simulink model "CoSimV1"  (R2025a)
settings: Solver=FixedStepDiscrete  StartTime=0.0  StopTime=1  FixedStep=Ts_Power  MaxStep=1e-7  RelTol=1e-4  EnableMultiTasking=on
PreLoadFcn:
  | CosimInit
values from neighbouring files (symbols this model uses):
  C_PFC = 2600e-6    (= 0.0026)    [CosimInit.m]
  estimation_src = 3    [CosimInit.m]
  Fnom = 50    [CosimInit.m]
  Fr_I = Fnom*2    (= 100)    [CosimInit.m]
  Ki_V = 80    [CosimInit.m]
  Kp_I = 0.06    [CosimInit.m]
  Kp_V = 0.25    [CosimInit.m]
  Kr_I = 2.5    [CosimInit.m]
  L_PFC = 600e-6    (= 0.0006)    [CosimInit.m]
  Limit_V = 100    [CosimInit.m]
  mm_10cycle_points = mm_points_per_cycle * 10    (= 800)    [CosimInit.m]
  mm_fund_freq = 50    [CosimInit.m]
  mm_points_per_cycle = 80    [CosimInit.m]
  RL_PFC = 20e-3    (= 0.02)    [CosimInit.m]
  Ro = 22.22    [CosimInit.m]
  Ts_Control = 1/Fc    (= 5e-05)    [CosimInit.m]
  Ts_Power = 50e-9    (= 5e-08)    [CosimInit.m]
  use_d_predict = 1    [CosimInit.m]
  use_harmonic = 1    [CosimInit.m]
  use_p_predict = 0    [CosimInit.m]
  Vnom_ac = 240    [CosimInit.m]
undefined symbols (not defined in the file or in its folder): DiscIntNeverNeededParam
libraries: spsSeriesRLCBranchLib x4, spsMeanLib x4, spsCurrentMeasurementLib x3, spsDiodeLib x2, MyLibrary x2, spsFourierLib x2, spsTHDLib x2, pycoexlib x2, simulink x2, spsVoltageMeasurementLib x2, spsACVoltageSourceLib x1, spsIdealSwitchLib x1
settings Model: SimulationMode=accelerator  Creator=The MathWorks, Inc.  LastModifiedBy=changhong
settings SolverCC: AlgebraicLoopSolver=TrustRegion  SolverResetMethod=Robust  AutoInsertRateTranBlk=on
settings DataIOCC: SaveOutput=off  SignalLogging=off  DSMLogging=off  SaveTime=off  ReturnWorkspaceOutputs=off
settings OptimizationCC: LifeSpan=inf
settings DebuggingCC: UnconnectedInputMsg=warning  UnconnectedOutputMsg=warning  UnconnectedLineMsg=warning  SFUnexpectedBacktrackingDiag=warning  SFNoUnconditionalDefaultTransitionDiag=warning  SFExecutionAtInitializationDiag=none  ArithmeticOperatorsInVariantConditions=warning
settings ModelReferenceCC: EnableRefExpFcnMdlSchedulingChecks=on
settings SFSimCC: SimUseLocalCustomCode=off  CustomCodeUndefinedFunction=UseInterfaceOnly
settings RTWCC: RTWUseLocalCustomCode=off  GPUComputeCapability=3.5  DLArmComputeVersion=19.05
settings CodeAppCC: StateflowObjectComments=on
settings GRTTargetCC: TargetLangStandard=C89/C90 (ANSI)
settings ConfigComp: CovMetricSettings=dw  CovSaveCumulativeToWorkspaceVar=on  CovSaveSingleToWorkspaceVar=on  CovExternalEMLEnable=off
settings SimscapeCC: SimscapeNormalizeSystem=off  SimscapeNominalValues={1, 'bar'; 1, 'cm^3/s'; 1, 'bar*kg/s'; 1, 'kJ/kg'; 1, 'kW'; }

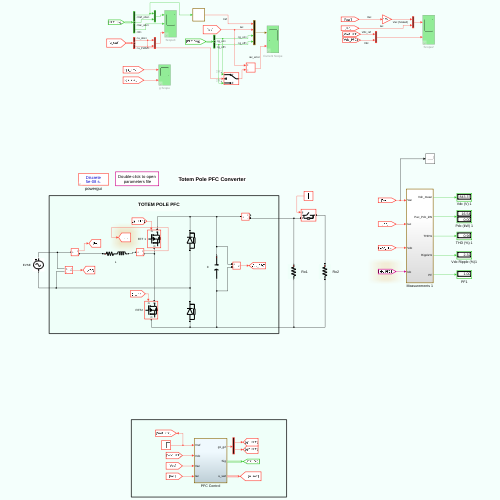
[thumbnail: Simulink's stored preview of the top-level diagram]
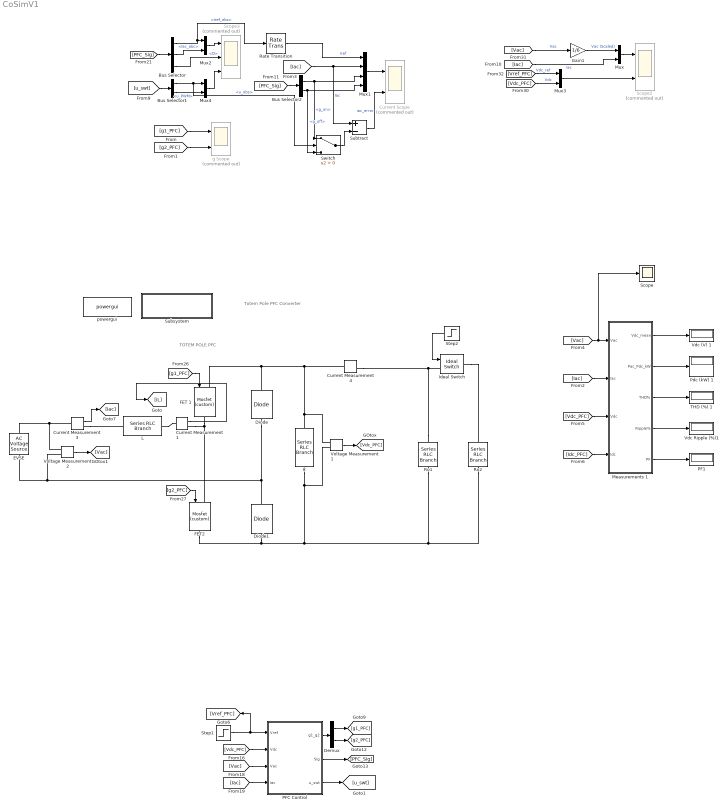
== system CoSimV1 ==
  note: Totem Pole PFC Converter
  note: TOTEM POLE PFC
  Bus Selector : BusSelector  OutputSignals=Iref_obs,Iac_abc,D
  Bus Selector1 : BusSelector  OutputSignals=u_obs,u_PWM
  Bus Selector2 : BusSelector  OutputSignals=g_on,g_off
  C : spsSeriesRLCBranchLib/Series RLC Branch  LConnTagsString=__new0  RConnTagsString=__new0  BranchType=C  Resistance=1  Inductance=1e-3  SetiL0=off  InitialCurrent=0  Capacitance=C_PFC  Setx0=on  InitialVoltage=375  Measurements=None
  Current Measurement1 : spsCurrentMeasurementLib/Current Measurement  PhasorSimulation=off  OutputType=Complex  PSBequivalent=0
  Current Measurement3 : spsCurrentMeasurementLib/Current Measurement  PhasorSimulation=off  OutputType=Complex  PSBequivalent=0
  Current Measurement4 : spsCurrentMeasurementLib/Current Measurement  PhasorSimulation=off  OutputType=Complex  PSBequivalent=0
  Current Scope : Scope  Commented=on  NumInputPorts=2
      settings: ActiveDisplayYMinimum=-76.387109863432016  ActiveDisplayYMaximum=79.51420484932207  DataLoggingVariableName=ScopeData3
  Demux : Demux  Outputs=2
  Diode : spsDiodeLib/Diode  Ron=Ron_Diode  Lon=0  Vf=Vf  IC=0  UseSnubber=0  Rs=1e6  Cs=inf  Measurements=off
  Diode1 : spsDiodeLib/Diode  Ron=Ron_Diode  Lon=0  Vf=Vf  IC=0  UseSnubber=0  Rs=1e6  Cs=inf  Measurements=off
  EVSE : spsACVoltageSourceLib/AC Voltage Source  Amplitude=Vnom_ac*sqrt(2)  Phase=0  Frequency=Fnom  SampleTime=Ts_Power  Measurements=None  BusType=swing  Pref=10e3  Qref=0  Qmin=-inf  Qmax=+inf
  FET 1 : MyLibrary/Mosfet (custom)  Ron=Ron_FET  Lon=0  Rd=Ron_Diode  Vfd=Vf  IC=0  Rs=1e6  Cs=inf  Measurements=off
  FET2 : MyLibrary/Mosfet (custom)  Ron=Ron_FET  Lon=0  Rd=Ron_Diode  Vfd=Vf  IC=0  Rs=1e6  Cs=inf  Measurements=off
  Gain1 : Gain  Gain=1/6
  Ideal Switch : spsIdealSwitchLib/Ideal Switch  Ron=0.001  Lon=0  IC=0  Rs=1e5  Cs=inf  Measurements=off
  L : spsSeriesRLCBranchLib/Series RLC Branch  LConnTagsString=__new0  RConnTagsString=__new0  BranchType=RL  Resistance=RL_PFC  Inductance=L_PFC  SetiL0=off  InitialCurrent=0  Capacitance=1e-6  Setx0=off  InitialVoltage=0  Measurements=None
  Measurements 1 : Subsystem
  Mux{,2..4} (4 alike) : Mux  Inputs=2
  Mux1 : Mux
  PF1 : Display
      settings: Format=bank  Decimation=100
  PFC Control : Subsystem
  Pdc (kW) 1 : Display
      settings: Format=bank  Decimation=100
  Rate Transition : RateTransition
  Ro1 : spsSeriesRLCBranchLib/Series RLC Branch  LConnTagsString=__new0  RConnTagsString=__new0  BranchType=R  Resistance=Ro*2  Inductance=200e-6  SetiL0=off  InitialCurrent=0  Capacitance=400e-6  Setx0=off  InitialVoltage=0  Measurements=None
  Ro2 : spsSeriesRLCBranchLib/Series RLC Branch  LConnTagsString=__new0  RConnTagsString=__new0  BranchType=R  Resistance=Ro*2  Inductance=200e-6  SetiL0=off  InitialCurrent=0  Capacitance=400e-6  Setx0=off  InitialVoltage=0  Measurements=None
  Scope : Scope
      settings: DataLoggingVariableName=ScopeData7
  Scope2 : Scope  Commented=on  NumInputPorts=2
      settings: ActiveDisplayYMinimum=-127.22187930583854  ActiveDisplayYMaximum=127.21088523305926  DataLoggingVariableName=ScopeData11
  Scope3 : Scope  Commented=on  NumInputPorts=3
      settings: ActiveDisplayYMinimum=-13.42740578837777  ActiveDisplayYMaximum=110.84665209539996  DataLoggingVariableName=ScopeData2
  Step1 : Step  Time=0.2  Before=350  After=400  SampleTime=Ts_Power
  Step2 : Step  Time=0.4  SampleTime=Ts_Power
  Subsystem : Subsystem
      settings: OpenFcn=edit('Totem_Pole_PFC_v1_data');
      mask Display: disp('Double-click to open\n parameters file');
  Subtract : Sum  Inputs=+-
  Switch : Switch  Criteria=u2 > Threshold  SaturateOnIntegerOverflow=off  InputSameDT=off
  THD (%) 1 : Display
      settings: Format=bank  Decimation=100
  Vdc (V) 1 : Display
      settings: Format=bank  Decimation=100
  Vdc Ripple (%)1 : Display
      settings: Format=bank  Decimation=100
  Voltage Measurement1 : spsVoltageMeasurementLib/Voltage Measurement  PhasorSimulation=off  OutputType=Complex  PSBequivalent=0
  Voltage Measurement2 : spsVoltageMeasurementLib/Voltage Measurement  PhasorSimulation=off  OutputType=Complex  PSBequivalent=0
  g Scope : Scope  Commented=on  NumInputPorts=2
      settings: ActiveDisplayYMinimum=-0.12499999999999997  ActiveDisplayYMaximum=1.125
  powergui : spspowerguiLib/powergui  Priority=1  SimulationMode=Discrete  SampleTime=Ts_Power  frequency=60  Iterations=50  frequencyindice=0  Pbase=100e6  ErrMax=1e-4  UnitsV=kV  UnitsW=MW  buscounter=0  FunctionMessages=off  echomessages=off  EnableUseOfTLC=off  CurrentSourceSwitches=off  DisableSnubberDevices=off  DisableRonSwitches=off  DisableVfSwitches=off  DisplayEquations=off  AutomaticDiscreteSolvers=off  SolverType=Tustin/Backward Euler (TBE)  Interpol=off  ExternalGateDelay=off  methode=off  Ts=100  x0status=blocks  SPID=on  SwTol=0  HookPort=off  NonlinearTolerance=1e-4  nMaxIteration=100  ContinueOnMaxIteration=off  RestoreLinks=warning  ResistiveCurrentMeasurement=off  Frange=[0:2:500]  Ylog=off  Xlog=on  ShowGrid=off  save=off  variable=ZData  structure=0  ZoomFFT=off  StartTime=0.0  cycles=1  DisplayStyle=1  fundamental=60  FreqAxis=off  MaxFrequency=1000  frequencyindicesteady=1  RmsSteady=1  display=off
  wires:
  Current Measurement3/1 -> [Iac]
  [g1_PFC] -> FET 1/1
  [g2_PFC] -> FET2/1
  Voltage Measurement1/1 -> [Vdc_PFC]
  Step2/1 -> Ideal Switch/1
  Voltage Measurement2/1 -> [Vac]
  Current Measurement1/1 -> [iL]
  Step1/1 -> PFC Control/1(Vref), [Vref_PFC]
  Demux/1 -> [g1_PFC]
  Demux/2 -> [g2_PFC]
  Switch/1 -> Subtract/2
  Bus Selector/1 -> Rate Transition/1, Mux2/1  "<Iref_obs>"
  Rate Transition/1 -> Mux1/1  "Iref"
  Bus Selector1/1 -> Mux4/1, Switch/2  "<u_obs>"
  Bus Selector/2 -> Mux2/2  "<Iac_abc>"
  Mux3/1 -> Scope2/2
  Mux/1 -> Scope2/1
  [g2_PFC] -> g Scope/2
  Bus Selector2/2 -> Mux1/4, Switch/3  "<g_off>"
  Measurements 1/5(PF) -> PF1/1
  [Idc_PFC] -> Measurements 1/4(Idc)
  Bus Selector1/2 -> Mux4/2  "<u_PWM>"
  [Vac] -> Gain1/1  "Vac"
  Measurements 1/2(Pac_Pdc_kW) -> Pdc (kW) 1/1
  Bus Selector/3 -> Scope3/2  "<D>"
  Measurements 1/4(Ripple%) -> Vdc Ripple (%)1/1
  [u_swt] -> Bus Selector1/1
  Mux1/1 -> Current Scope/1
  Gain1/1 -> Mux/1  "Vac (Scaled)"
  [PFC_Sig] -> Bus Selector2/1
  [g1_PFC] -> g Scope/1
  [Vdc_PFC] -> Measurements 1/3(Vdc)
  Measurements 1/3(THD%) -> THD (%) 1/1
  [Iac] -> Subtract/1, Mux1/2  "Iac"
  [Vac] -> Scope/1, Measurements 1/1(Vac)
  [Iac] -> Mux/2  "Iac"
  [PFC_Sig] -> Bus Selector/1
  Measurements 1/1(Vdc_mean) -> Vdc (V) 1/1
  [Iac] -> Measurements 1/2(Iac)
  Bus Selector2/1 -> Switch/1, Mux1/3  "<g_on>"
  Mux2/1 -> Scope3/1
  [Vref_PFC] -> Mux3/1  "Vdc_ref"
  [Vdc_PFC] -> Mux3/2  "Vdc"
  Mux4/1 -> Scope3/3
  Subtract/1 -> Current Scope/2  "iac_error"
  [Vdc_PFC] -> PFC Control/2(Vdc)
  [Vac] -> PFC Control/3(Vac)
  [Iac] -> PFC Control/4(Iac)
  PFC Control/1(g1_g2) -> Demux/1
  PFC Control/2(Sig) -> [PFC_Sig]
  PFC Control/3(u_swt) -> [u_swt]
  connections:
  Ro1/RConn1 -- C/RConn1 -- Voltage Measurement1/LConn2 -- FET2/RConn1 -- Diode1/LConn1 -- Ro2/RConn1
  FET2/LConn1 -- FET 1/RConn1 -- Current Measurement1/RConn1
  EVSE/LConn1 -- Diode/LConn1 -- Diode1/RConn1 -- Voltage Measurement2/LConn2
  Diode/RConn1 -- FET 1/LConn1 -- Voltage Measurement1/LConn1 -- C/LConn1 -- Current Measurement4/LConn1
  Ro1/LConn1 -- Current Measurement4/RConn1 -- Ideal Switch/LConn1
  EVSE/RConn1 -- Current Measurement3/LConn1 -- Voltage Measurement2/LConn1
  L/RConn1 -- Current Measurement1/LConn1
  Current Measurement3/RConn1 -- L/LConn1
  Ideal Switch/RConn1 -- Ro2/LConn1

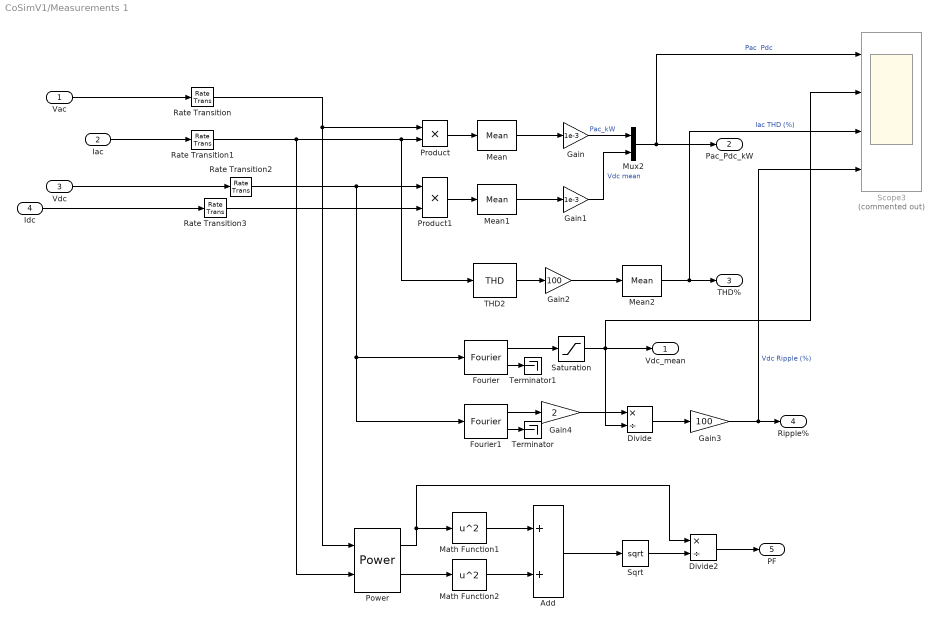
== system CoSimV1/Measurements 1 ==
  Vac : Inport
  Iac : Inport  Port=2
  Vdc : Inport  Port=3
  Idc : Inport  Port=4
  Add : Sum
  Divide : Product  Inputs=*/
  Divide2 : Product  Inputs=*/
  Fourier : spsFourierLib/Fourier  Freq=Fnom  n=0  InInit=[0, 0]  Ts=Ts_Control
  Fourier1 : spsFourierLib/Fourier  Freq=Fnom  n=2  InInit=[0, 0]  Ts=Ts_Control
  Gain : Gain  Gain=1e-3
  Gain1 : Gain  Gain=1e-3
  Gain2 : Gain  Gain=100
  Gain3 : Gain  Gain=100
  Gain4 : Gain  Gain=2
  Math Function1 : Math  Operator=square
  Math Function2 : Math  Operator=square
  Mean : spsMeanLib/Mean  Freq=Fnom  Vinit=0  Ts=Ts_Control
  Mean1 : spsMeanLib/Mean  Freq=Fnom  Vinit=0  Ts=Ts_Control
  Mean2 : spsMeanLib/Mean  Freq=Fnom  Vinit=0  Ts=Ts_Control
  Mux2 : Mux  Inputs=2
  Power : spsPowerLib/Power  Freq=Fnom  Vinit=[1, 0]  Iinit=[1, 0]  Ts=Ts_Control
  Product : Product
  Product1 : Product
  Rate Transition{,1..3} (4 alike) : RateTransition  OutPortSampleTime=Ts_Control
  Saturation : Saturate  UpperLimit=inf  LowerLimit=eps
  Scope3 : Scope  Commented=on  NumInputPorts=4
      settings: ActiveDisplayYMinimum=-1.32447  ActiveDisplayYMaximum=11.92024
  Sqrt : Sqrt
  THD2 : spsTHDLib/THD  Freq=Fnom  Ts=Ts_Control
  Terminator : Terminator
  Terminator1 : Terminator
  Vdc_mean : Outport
  Pac_Pdc_kW : Outport  Port=2
  THD% : Outport  Port=3
  Ripple% : Outport  Port=4
  PF : Outport  Port=5
  wires:
  Gain1/1 -> Mux2/2  "Vdc mean"
  Product1/1 -> Mean1/1
  Mean/1 -> Gain/1
  Product/1 -> Mean/1
  Gain/1 -> Mux2/1  "Pac_kW"
  THD2/1 -> Gain2/1
  Mean1/1 -> Gain1/1
  Iac/1 -> Rate Transition1/1
  Mux2/1 -> Scope3/1, Pac_Pdc_kW/1  "Pac  Pdc"
  Gain2/1 -> Mean2/1
  Mean2/1 -> Scope3/3, THD%/1  "Iac THD (%)"
  Fourier/2 -> Terminator1/1
  Fourier/1 -> Saturation/1
  Saturation/1 -> Scope3/2, Vdc_mean/1, Divide/2
  Divide/1 -> Gain3/1
  Fourier1/1 -> Gain4/1
  Gain4/1 -> Divide/1
  Fourier1/2 -> Terminator/1
  Gain3/1 -> Scope3/4, Ripple%/1  "Vdc Ripple (%)"
  Power/1 -> Math Function1/1, Divide2/1
  Power/2 -> Math Function2/1
  Math Function1/1 -> Add/1
  Math Function2/1 -> Add/2
  Add/1 -> Sqrt/1
  Sqrt/1 -> Divide2/2
  Divide2/1 -> PF/1
  Rate Transition1/1 -> Power/2, THD2/1, Product/2
  Vdc/1 -> Rate Transition2/1
  Idc/1 -> Rate Transition3/1
  Rate Transition/1 -> Power/1, Product/1
  Vac/1 -> Rate Transition/1
  Rate Transition2/1 -> Product1/1, Fourier/1, Fourier1/1
  Rate Transition3/1 -> Product1/2

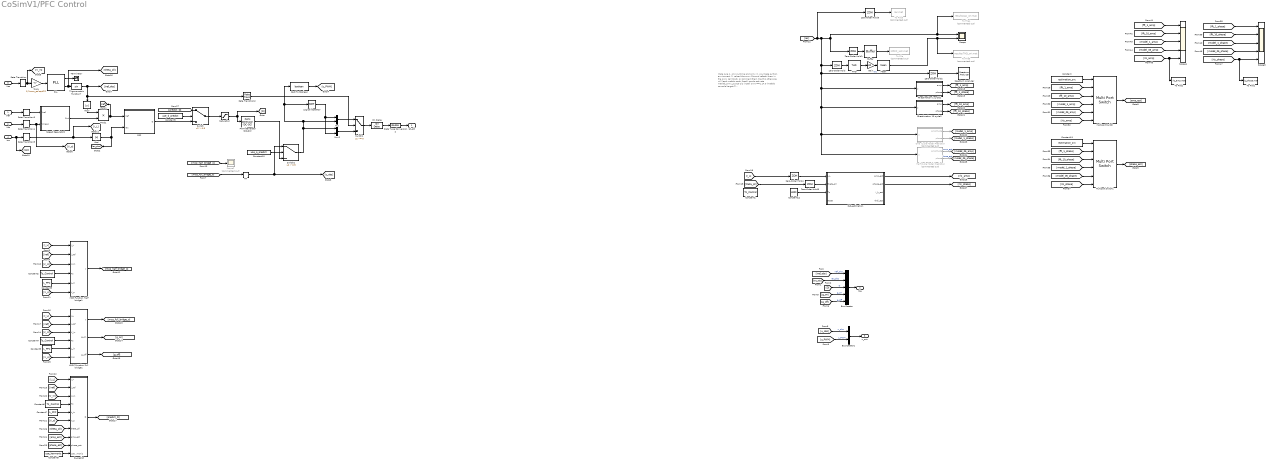
== system CoSimV1/PFC Control ==
  note: Make sure
      | 1. onnxruntime and onnx in your base python enviroment.
      | 2. reload the onnx file and refresh them in the onnx call block.
      | or comment them like this
      | otherwise will lead matlab crash
      |
      | (bash)
      | conda activate matlab_onnx_py310
      | pip install onnx==1.14.0
      |
      | (matlab console)
      | target = "/home/changhong/anaconda3/envs/matlab_onnx_py310/bin/python";
      | pe = pyenv
      | pyenv("Version", target)
  Vref : Inport
  Vdc : Inport  Port=2
  Vac : Inport  Port=3
  Iac : Inport  Port=4
  AbsI : Abs  SaturateOnIntegerOverflow=off
  AbsV : Abs  SaturateOnIntegerOverflow=off
  Buffer : Buffer  N=80  V=79  OutputFrames=off
  Bus Creator : BusCreator  Inputs=5
  Bus Creator1 : BusCreator  Inputs=2
  Cast To Boolean : DataTypeConversion  OutDataTypeStr=boolean  SaturateOnIntegerOverflow=off  RndMeth=Floor
  Constant : Constant  Value=estimation_src
  Constant{1..2,4,6} (4 alike) : Constant  Value=Ts_Control
  Constant10 : Constant  Value=use_p_predict
  Constant11 : Constant  Value=estimation_src
  Constant12 : Constant  Value=4000
  Constant3 : Constant  Value=L_PFC
  Constant5 : Constant  Value=L_PFC
  Constant7 : Constant  Value=L_PFC
  Constant8 : Constant  Value=use_harmonic
  Constant9 : Constant  Value=use_d_predict
  D_predict : MATLAB Function  TreatAsAtomicUnit=on
  Data Type Conversion2 : DataTypeConversion  OutDataTypeStr=double  SaturateOnIntegerOverflow=off  RndMeth=Floor
  Gain : Gain  Gain=100
  Half Cycle Model Prediction : Subsystem  Commented=on
  Logical Operator : Logic  Operator=NOT  AllPortsSameDT=off  OutDataTypeStr=float('double')
  MCP Function Half bridge1 : MATLAB Function  TreatAsAtomicUnit=on
  Mean : spsMeanLib/Mean  Freq=50  Vinit=0  Ts=1/4000
  Multiport Switch : MultiPortSwitch  Inputs=5  SaturateOnIntegerOverflow=off  InputSameDT=off
  Multiport Switch1 : MultiPortSwitch  Inputs=5  SaturateOnIntegerOverflow=off  InputSameDT=off
  Mux : Mux  Inputs=2
  Mux2 : Mux  Inputs=2
  On Delay : spsOnDelayLib/On Delay  DelayType=On delay  delay=DT_PFC  ic=0  Ts=Ts_Power
  One  Cycle Model Prediction : Subsystem  Commented=on
  PLL : spsPLLLib/PLL  Fmin=0.9*Fnom  Par_Init=[0, Fnom]  ParK=[180, 3200, 1]  TcD=1e-4  MaxRateChangeFreq=12  FilterCutOffFreq=25  Ts=Ts_Control  AGC=on
  PR2 : Subsystem  mask(Current Regulator (Pr)){Kp=Kp_I, Kr=Kr_I, Fr=Fr_I}
      mask prompts: Kp "Proportional gain"; Kr "Resonant gain"; Fr "Resonant frequency (Hz)"
      mask help: This block implements a currentregulator using a PR controller.
      mask Display: disp('Current Regulator\n PR');
  PWM Generator (DC-DC) : spsPWMGeneratorDCDCLib/PWM Generator (DC-DC)  Fsw=Fsw  Ts=Ts_Power
  Prod1 : Product
  RLS_estimation : MATLAB Function  TreatAsAtomicUnit=on
  RT : RateTransition  OutPortSampleTime=5e-08
  Rate Transition{,3..5} (4 alike) : RateTransition  OutPortSampleTime=Ts_Control
  Rate Transition2 : RateTransition  OutPortSampleTime=Ts_Power
  Saturation : Saturate  UpperLimit=1  LowerLimit=0
  Scope : Scope  NumInputPorts=2
      settings: ActiveDisplayYMinimum=-211.21899325155135  ActiveDisplayYMaximum=223.70734437609497  DataLoggingVariableName=ScopeData4
  Scope1 : Scope  NumInputPorts=5
      settings: ActiveDisplayYMinimum=-19.486412563330539  ActiveDisplayYMaximum=175.37771306999088  DataLoggingVariableName=ScopeData5
  Scope2 : Scope  Commented=on
      settings: DataLoggingVariableName=ScopeData9
  Scope3 : Scope  NumInputPorts=5
      settings: ActiveDisplayYMinimum=-3.9269908169872414  ActiveDisplayYMaximum=3.926990816987241  DataLoggingVariableName=ScopeData6
  Spectrum Analyzer : SpectrumAnalyzer  WindowPosition=[1761.000000,30.000000,1850.000000,1136.000000,]  ScopeFrameLocation=window  SampleRateSource=Property  SampleRate=8000  PlotAsTwoSidedSpectrum=off  WindowInvariantSamplesPerUpdate=on  FrequencySpan=Start and stop frequencies  StartFrequency=0  StopFrequency=2000  YLimits=[1.4645 59.0786]  ColorLimits=[-42.4528 59.157]
  Speed Regulator2 : Subsystem  DialogController=POWERSYS.PowerSysDialog  mask(Voltage Regulator){Kp=Kp_V, Ki=Ki_V, Limit_wreg=Limit_V, Init=0, Ts=Ts_Control}
      mask prompts: Kp "Proportional gain (Kp):"; Ki "Integral gain (Ki):"; Limit_wreg "Output limits"; Init "Output initial value:"; Ts "Sample time:"
      mask help: This block implements a voltage regulator using an ant-windup PI controller.
      mask Display: disp('Voltage\nRegulator');
  Switch : Switch  Criteria=u2 > Threshold  Threshold=0.5  SaturateOnIntegerOverflow=off  InputSameDT=off
  Switch1 : Switch  SaturateOnIntegerOverflow=off  InputSameDT=off
  Switch2 : Switch  Criteria=u2 > Threshold  Threshold=0.5  SaturateOnIntegerOverflow=off  InputSameDT=off
  THD : spsTHDLib/THD  Freq=50  Ts=1/4000
  Terminator : Terminator
  To File : ToFile  Commented=on  Filename=MPCC_IAC.mat  SaveFormat=Timeseries
  To File1 : ToFile  Filename=rls_phase.mat  SaveFormat=Timeseries
  To File2 : ToFile  Filename=rls_amp.mat  SaveFormat=Timeseries
  To File3 : ToFile  Commented=on  Filename=Iac.mat  SaveFormat=Timeseries
  To File4 : ToFile  Commented=on  Filename=results/Iac_ori.mat  SaveFormat=Timeseries
  To File5 : ToFile  Commented=on  Filename=results/THD_ori.mat  SaveFormat=Timeseries
  Trigonometric Function7 : Trigonometry
  UMPC Function Full bridge1 : MATLAB Function  TreatAsAtomicUnit=on
  Zero-Order Hold{,1,3..5} (5 alike) : ZeroOrderHold  SampleTime=1/4000
  Zero-Order Hold2 : ZeroOrderHold  SampleTime=1/8000
  fft estimation 1 cycle2 : Subsystem
  fft estimation 10 cycle2 : Subsystem
  to-pu : Gain  Gain=1/(Vnom_ac*sqrt(2))
  g1_g2 : Outport  PortDimensions=2
  Sig : Outport  Port=2
  u_swt : Outport  Port=3
  wires:
  Mux/1 -> Switch1/1
  Iac/1 -> [Iac], Rate Transition5/1
  Speed Regulator2/1(Out) -> Prod1/2
  Rate Transition2/1 -> Switch1/2
  Data Type Conversion2/1 -> g1_g2/1
  PLL/2 -> [theta_pll], Trigonometric Function7/1
  Saturation/1 -> PWM Generator (DC-DC)/1, [D]
  to-pu/1 -> PLL/1
  Rate Transition/1 -> [V_in], to-pu/1
  Bus Creator1/1 -> u_swt/1
  AbsI/1 -> PR2/2(Iac), [Iac_abs]
  Trigonometric Function7/1 -> AbsV/1, Rate Transition2/1, [Iref_obs]
  [D] -> Bus Creator/3  "D"
  Rate Transition3/1 -> Speed Regulator2/1(Vref)
  Switch1/1 -> On Delay/1
  Rate Transition4/1 -> Speed Regulator2/2(Vmeas), [V_o]
  [u_obs] -> Bus Creator1/1  "u_obs"
  Mux2/1 -> Switch1/3
  Vdc/1 -> Rate Transition4/1
  [mcp_full_bridge_o] -> RT/1
  [Iref_obs] -> Bus Creator/1  "Iref_obs"
  RT/1 -> Switch2/1, [u_obs]
  Cast To Boolean/1 -> [u_PWM]
  PWM Generator (DC-DC)/1 -> Switch2/3
  Vac/1 -> Rate Transition/1
  Prod1/1 -> [Iref], PR2/1(Iref)
  Bus Creator/1 -> Sig/1
  Rate Transition5/1 -> [i_L], AbsI/1
  PLL/1 -> Terminator/1
  AbsV/1 -> Prod1/1
  [Iac_abs] -> Bus Creator/2  "Iac_abc"
  Switch2/1 -> Logical Operator/1, Cast To Boolean/1, Mux/2, Mux2/1
  Vref/1 -> Rate Transition3/1
  On Delay/1 -> Data Type Conversion2/1
  [u_PWM] -> Bus Creator1/2  "u_PWM"
  [Iac] -> Zero-Order Hold3/1, Half Cycle Model Prediction/1(u), One  Cycle Model Prediction/1(u), fft estimation 10 cycle2/1(u), fft estimation 1 cycle2/1(u), Zero-Order Hold2/1, Zero-Order Hold/1, Zero-Order Hold1/1, To File4/1, Scope/1  "Iac"
  Buffer/1 -> To File/1
  Gain/1 -> Mean/1
  Zero-Order Hold/1 -> THD/1
  Mean/1 -> To File5/1, Scope/2
  Zero-Order Hold2/1 -> Spectrum Analyzer/1
  THD/1 -> Gain/1
  Zero-Order Hold1/1 -> Buffer/1
  [i_L] -> MCP Function Half bridge1/1(i_L)
  [Iref] -> MCP Function Half bridge1/2(i_ref)
  [V_in] -> MCP Function Half bridge1/3(V_in)
  Constant2/1 -> MCP Function Half bridge1/4(Ts)
  Constant3/1 -> MCP Function Half bridge1/5(L_in)
  [V_o] -> MCP Function Half bridge1/6(V_o)
  MCP Function Half bridge1/1(y) -> [mcp_half_bridge_o]
  [i_L] -> UMPC Function Full bridge1/1(i_L)
  [Iref] -> UMPC Function Full bridge1/2(i_ref)
  [V_in] -> UMPC Function Full bridge1/3(V_in)
  Constant4/1 -> UMPC Function Full bridge1/4(Ts)
  Constant5/1 -> UMPC Function Full bridge1/5(L_in)
  [V_o] -> UMPC Function Full bridge1/6(V_o)
  UMPC Function Full bridge1/1(y) -> [mcp_full_bridge_o]
  UMPC Function Full bridge1/2(g_on) -> [g_on]
  UMPC Function Full bridge1/3(g_off) -> [g_off]
  [g_on] -> Bus Creator/4  "g_on"
  [g_off] -> Bus Creator/5  "g_off"
  [theta_pll] -> Zero-Order Hold5/1
  [i_L] -> D_predict/1(i_L)
  [Iref] -> D_predict/2(i_ref)
  [V_in] -> D_predict/3(V_in)
  Constant6/1 -> D_predict/4(Ts)
  Constant7/1 -> D_predict/5(L_in)
  [V_o] -> D_predict/6(V_o)
  [amp_est] -> D_predict/8(amp_est)
  [phase_est] -> D_predict/9(phase_est)
  Constant8/1 -> D_predict/10(use_harmonic)
  [theta_pll] -> D_predict/7(theta_pll)
  D_predict/1(D) -> [predict_D]
  [mcp_half_bridge_o] -> Scope2/1
  Constant9/1 -> Switch/2
  [predict_D] -> Switch/1
  PR2/1(D) -> Switch/3
  Switch/1 -> Saturation/1
  Constant10/1 -> Switch2/2
  Logical Operator/1 -> Mux2/2, Mux/1
  Constant/1 -> Multiport Switch/1
  fft estimation 1 cycle2/1(amp) -> [fft_1_amp]
  fft estimation 1 cycle2/2(phase) -> [fft_1_phase]
  fft estimation 10 cycle2/1(amp) -> [fft_10_amp]
  fft estimation 10 cycle2/2(phase) -> [fft_10_phase]
  One  Cycle Model Prediction/1(amplitude) -> [model_1_amp]
  One  Cycle Model Prediction/2(phase) -> [model_1_phase]
  Half Cycle Model Prediction/1(amplitude) -> [model_05_amp]  "amp_est"
  Half Cycle Model Prediction/2(phase) -> [model_05_phase]  "hase_est"
  Multiport Switch/1 -> [amp_est]
  RLS_estimation/1(amp_est) -> [rls_amp]
  RLS_estimation/2(phase_est) -> [rls_phase]
  [fft_1_amp] -> Multiport Switch/2
  [fft_10_amp] -> Multiport Switch/3
  [model_1_amp] -> Multiport Switch/4
  [model_05_amp] -> Multiport Switch/5
  [rls_amp] -> Multiport Switch/6
  [rls_phase] -> Multiport Switch1/6
  [model_05_phase] -> Multiport Switch1/5
  [model_1_phase] -> Multiport Switch1/4
  [fft_10_phase] -> Multiport Switch1/3
  [fft_1_phase] -> Multiport Switch1/2
  Multiport Switch1/1 -> [phase_est]
  Constant11/1 -> Multiport Switch1/1
  [fft_1_amp] -> Scope1/1
  [fft_10_amp] -> Scope1/2
  [model_1_amp] -> Scope1/3
  [model_05_amp] -> Scope1/4
  [rls_amp] -> To File2/1, Scope1/5
  [fft_1_phase] -> Scope3/1
  [fft_10_phase] -> Scope3/2
  [model_1_phase] -> Scope3/3
  [model_05_phase] -> Scope3/4
  [rls_phase] -> To File1/1, Scope3/5
  Zero-Order Hold3/1 -> To File3/1
  [i_L] -> Zero-Order Hold4/1
  Constant12/1 -> RLS_estimation/3(Ts)
  Zero-Order Hold4/1 -> RLS_estimation/1(i_L)
  Zero-Order Hold5/1 -> RLS_estimation/2(theta_pll)

== system CoSimV1/Subsystem ==

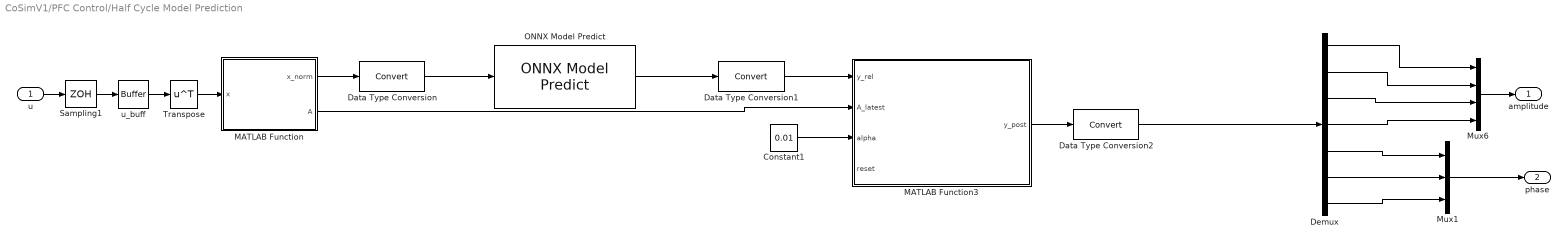
== system CoSimV1/PFC Control/Half Cycle Model Prediction ==
  u : Inport
  Constant1 : Constant  Value=0.01
  Data Type Conversion : DataTypeConversion  SaturateOnIntegerOverflow=off  RndMeth=Floor
  Data Type Conversion1 : DataTypeConversion  SaturateOnIntegerOverflow=off  RndMeth=Floor
  Data Type Conversion2 : DataTypeConversion  SaturateOnIntegerOverflow=off  RndMeth=Floor
  Demux : Demux  Outputs=7
  MATLAB Function : MATLAB Function  TreatAsAtomicUnit=on
  MATLAB Function3 : MATLAB Function  TreatAsAtomicUnit=on
  Mux1 : Mux  Inputs=3
  Mux6 : Mux
  ONNX Model Predict : pycoexlib/ONNX Model Predict  ModelFile=/home/changhong/prj/finn_cli_fork/scripts/HIL/HarmonicAI_Simulation/Model_Training2/harmonic_brevitas_run_half_opt/brevitas_harmonic_mlp.onnx  ExecutionProviders=CPUExecutionProvider  InputTable={ 'input', 'float32', '', '2' }  OutputTable={ 'output', '', '' }  SampleTime=1/2000  InputDatatypes=float32  InputNumDims=2  InputPermutations=[]  OutputPermutations=[]  PythonCoexecutionBlockType=ONNXModelBlock  VariableOutputMaxSizes=[]
  Sampling1 : ZeroOrderHold  SampleTime=1/2000
  Transpose : Math  Operator=transpose
  u_buff : Buffer  N=40  V=39  OutputFrames=off
  amplitude : Outport
  phase : Outport  Port=2
  wires:
  Transpose/1 -> MATLAB Function/1(x)
  u_buff/1 -> Transpose/1
  u/1 -> Sampling1/1
  Mux1/1 -> phase/1
  Mux6/1 -> amplitude/1
  Data Type Conversion2/1 -> Demux/1
  MATLAB Function3/1(y_post) -> Data Type Conversion2/1
  Demux/1 -> Mux6/1
  Demux/2 -> Mux6/2
  Demux/3 -> Mux6/3
  Demux/4 -> Mux6/4
  Demux/5 -> Mux1/1
  Demux/6 -> Mux1/2
  Demux/7 -> Mux1/3
  MATLAB Function/2(A) -> MATLAB Function3/2(A_latest)
  Constant1/1 -> MATLAB Function3/3(alpha)
  Data Type Conversion1/1 -> MATLAB Function3/1(y_rel)
  ONNX Model Predict/1 -> Data Type Conversion1/1
  Data Type Conversion/1 -> ONNX Model Predict/1
  MATLAB Function/1(x_norm) -> Data Type Conversion/1
  Sampling1/1 -> u_buff/1

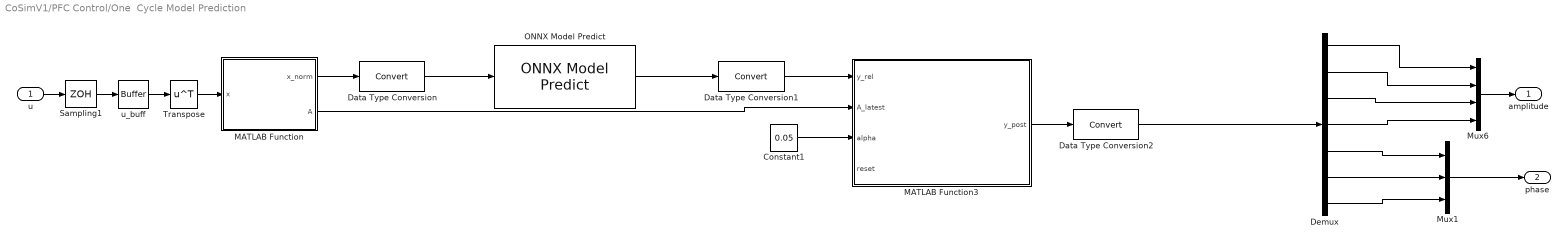
== system CoSimV1/PFC Control/One  Cycle Model Prediction ==
  u : Inport
  Constant1 : Constant  Value=0.05
  Data Type Conversion : DataTypeConversion  SaturateOnIntegerOverflow=off  RndMeth=Floor
  Data Type Conversion1 : DataTypeConversion  SaturateOnIntegerOverflow=off  RndMeth=Floor
  Data Type Conversion2 : DataTypeConversion  SaturateOnIntegerOverflow=off  RndMeth=Floor
  Demux : Demux  Outputs=7
  MATLAB Function : MATLAB Function  TreatAsAtomicUnit=on
  MATLAB Function3 : MATLAB Function  TreatAsAtomicUnit=on
  Mux1 : Mux  Inputs=3
  Mux6 : Mux
  ONNX Model Predict : pycoexlib/ONNX Model Predict  ModelFile=/home/changhong/prj/finn_cli_fork/scripts/HIL/HarmonicAI_Simulation/Model_Training2/harmonic_brevitas_run_1cycle/brevitas_harmonic_mlp.onnx  ExecutionProviders=AzureExecutionProvider, CPUExecutionProvider  InputTable={ 'input', 'float32', '', '2' }  OutputTable={ 'output', '', '' }  SampleTime=1/4000  InputDatatypes=float32  InputNumDims=2  InputPermutations=[]  OutputPermutations=[]  PythonCoexecutionBlockType=ONNXModelBlock  VariableOutputMaxSizes=[]
  Sampling1 : ZeroOrderHold  SampleTime=1/(mm_fund_freq*mm_points_per_cycle)
  Transpose : Math  Operator=transpose
  u_buff : Buffer  N=mm_points_per_cycle  V=mm_sampling_overlap  OutputFrames=off
  amplitude : Outport
  phase : Outport  Port=2
  wires:
  Sampling1/1 -> u_buff/1
  MATLAB Function/1(x_norm) -> Data Type Conversion/1
  Data Type Conversion/1 -> ONNX Model Predict/1
  ONNX Model Predict/1 -> Data Type Conversion1/1
  Data Type Conversion1/1 -> MATLAB Function3/1(y_rel)
  Constant1/1 -> MATLAB Function3/3(alpha)
  MATLAB Function/2(A) -> MATLAB Function3/2(A_latest)
  Demux/7 -> Mux1/3
  Demux/6 -> Mux1/2
  Demux/5 -> Mux1/1
  Demux/4 -> Mux6/4
  Demux/3 -> Mux6/3
  Demux/2 -> Mux6/2
  Demux/1 -> Mux6/1
  MATLAB Function3/1(y_post) -> Data Type Conversion2/1
  Data Type Conversion2/1 -> Demux/1
  Mux6/1 -> amplitude/1
  Mux1/1 -> phase/1
  u/1 -> Sampling1/1
  u_buff/1 -> Transpose/1
  Transpose/1 -> MATLAB Function/1(x)

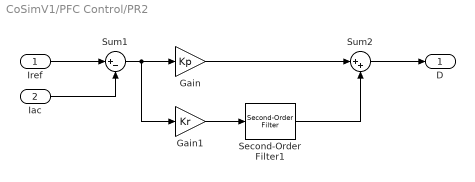
== system CoSimV1/PFC Control/PR2 ==
  Iref : Inport
  Iac : Inport  Port=2
  Gain : Gain  Gain=Kp
  Gain1 : Gain  Gain=Kr
  Second-Order Filter1 : spsSecondOrderFilterLib/Second-Order Filter  FilterType=Bandpass  Fo=Fr  Zeta=Zeta_I  Ts=Ts_Control  Initialize=off  Vac_Init="[0,  0,  60]"  Vdc_Init=0  PlotResponse=off  FreqRange=[0, 1000, 0.2]
  Sum1 : Sum  Inputs=|+-
  Sum2 : Sum  Inputs=|++
  D : Outport
  wires:
  Gain1/1 -> Second-Order Filter1/1
  Sum2/1 -> D/1
  Gain/1 -> Sum2/1
  Iac/1 -> Sum1/2
  Iref/1 -> Sum1/1
  Sum1/1 -> Gain1/1, Gain/1
  Second-Order Filter1/1 -> Sum2/2

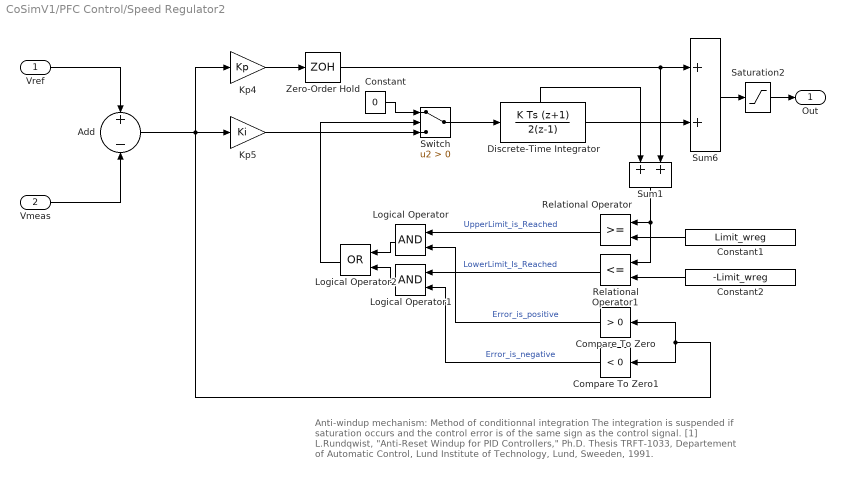
== system CoSimV1/PFC Control/Speed Regulator2 ==
  note: Anti-windup mechanism: Method of conditionnal integration
      |
      | The integration is suspended if saturation occurs and the
      | control error is of the same sign as the control signal.
      |
      | [1] L.Rundqwist, "Anti-Reset Windup for PID Controllers," Ph.D. Thesis TRFT-1033,
      | Departement of Automatic Control, Lund Institute of Technology, Lund, Sweeden, 1991.
  Vref : Inport  PortDimensions=1
  Vmeas : Inport  Port=2  PortDimensions=1
  Add : Sum  Inputs=+|-
  Compare To Zero : simulink/Logic and Bit Operations/Compare To Zero  relop=>  OutDataTypeStr=uint8  ZeroCross=off
  Compare To Zero1 : simulink/Logic and Bit Operations/Compare To Zero  relop=<  OutDataTypeStr=uint8  ZeroCross=off
  Constant : Constant  Value=0
  Constant1 : Constant  Value=Limit_wreg
  Constant2 : Constant  Value=-Limit_wreg
  Discrete-Time Integrator : DiscreteIntegrator  IntegratorMethod=Integration: Trapezoidal  InitialCondition=Init  SampleTime=Ts  LimitOutput=on  UpperSaturationLimit=Limit_wreg  LowerSaturationLimit=-Limit_wreg  ShowStatePort=on  ICPrevOutput=DiscIntNeverNeededParam  ICPrevScaledInput=DiscIntNeverNeededParam
  Kp4 : Gain  Gain=Kp  SaturateOnIntegerOverflow=on  SampleTime=Ts  OutDataTypeStr=Inherit: Same as input  ParamDataTypeStr=Inherit: Same as input
  Kp5 : Gain  Gain=Ki  SaturateOnIntegerOverflow=on  SampleTime=Ts  OutDataTypeStr=Inherit: Same as input  ParamDataTypeStr=Inherit: Same as input
  Logical Operator : Logic  AllPortsSameDT=off  OutDataTypeStr=boolean
  Logical Operator1 : Logic  AllPortsSameDT=off  OutDataTypeStr=boolean
  Logical Operator2 : Logic  Operator=OR  AllPortsSameDT=off  OutDataTypeStr=boolean
  Relational Operator : RelationalOperator  OutDataTypeStr=boolean  InputSameDT=off
  Relational Operator1 : RelationalOperator  Operator=<=  OutDataTypeStr=boolean  InputSameDT=off
  Saturation2 : Saturate  UpperLimit=Limit_wreg  LowerLimit=-Limit_wreg  SampleTime=Ts
  Sum1 : Sum  InputSameDT=on  SaturateOnIntegerOverflow=on  SampleTime=Ts  OutDataTypeStr=Inherit: Same as first input
  Sum6 : Sum  InputSameDT=on  SaturateOnIntegerOverflow=on  SampleTime=Ts  OutDataTypeStr=Inherit: Same as first input
  Switch : Switch  Criteria=u2 > Threshold  SaturateOnIntegerOverflow=off  InputSameDT=off
  Zero-Order Hold : ZeroOrderHold  SampleTime=Ts
  Out : Outport  SampleTime=Ts  InitialOutput=0  VectorParamsAs1DForOutWhenUnconnected=off
  wires:
  Kp5/1 -> Switch/3
  Switch/1 -> Discrete-Time Integrator/1
  Saturation2/1 -> Out/1
  Discrete-Time Integrator/1 -> Sum6/2
  Kp4/1 -> Zero-Order Hold/1
  Sum6/1 -> Saturation2/1
  Add/1 -> Compare To Zero/1, Compare To Zero1/1, Kp5/1, Kp4/1
  Compare To Zero1/1 -> Logical Operator1/2  "Error_is_negative"
  Logical Operator1/1 -> Logical Operator2/2
  Logical Operator/1 -> Logical Operator2/1
  Compare To Zero/1 -> Logical Operator/2  "Error_is_positive"
  Constant2/1 -> Relational Operator1/2
  Constant1/1 -> Relational Operator/2
  Relational Operator1/1 -> Logical Operator1/1  "LowerLimit_Is_Reached"
  Relational Operator/1 -> Logical Operator/1  "UpperLimit_is_Reached"
  Logical Operator2/1 -> Switch/2
  Sum1/1 -> Relational Operator/1, Relational Operator1/1
  Discrete-Time Integrator/State -> Sum1/1
  Zero-Order Hold/1 -> Sum6/1, Sum1/2
  Constant/1 -> Switch/1
  Vref/1 -> Add/1
  Vmeas/1 -> Add/2

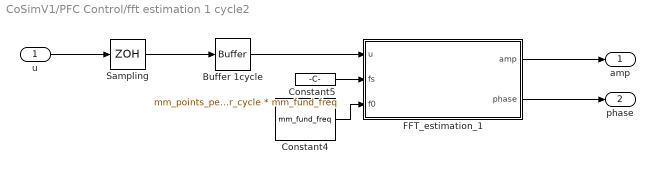
== system CoSimV1/PFC Control/fft estimation 1 cycle2 ==
  u : Inport
  Buffer 1cycle : Buffer  N=mm_points_per_cycle  V=mm_sampling_overlap  OutputFrames=off
  Constant4 : Constant  Value=mm_fund_freq
  Constant5 : Constant  Value=mm_points_per_cycle * mm_fund_freq
  FFT_estimation_1 : MATLAB Function  TreatAsAtomicUnit=on
  Sampling : ZeroOrderHold  SampleTime=1/(mm_fund_freq*mm_points_per_cycle)
  amp : Outport
  phase : Outport  Port=2
  wires:
  Sampling/1 -> Buffer 1cycle/1
  Buffer 1cycle/1 -> FFT_estimation_1/1(u)
  Constant5/1 -> FFT_estimation_1/2(fs)
  Constant4/1 -> FFT_estimation_1/3(f0)
  u/1 -> Sampling/1
  FFT_estimation_1/1(amp) -> amp/1
  FFT_estimation_1/2(phase) -> phase/1

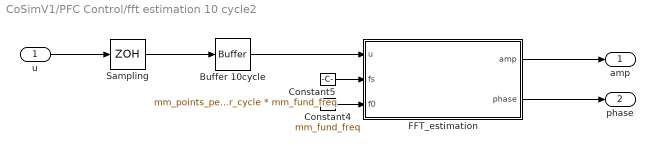
== system CoSimV1/PFC Control/fft estimation 10 cycle2 ==
  u : Inport
  Buffer 10cycle : Buffer  N=mm_10cycle_points  V=mm_10cycle_overlap  OutputFrames=off
  Constant4 : Constant  Value=mm_fund_freq
  Constant5 : Constant  Value=mm_points_per_cycle * mm_fund_freq
  FFT_estimation : MATLAB Function  TreatAsAtomicUnit=on
  Sampling : ZeroOrderHold  SampleTime=1/(mm_fund_freq*mm_points_per_cycle)
  amp : Outport
  phase : Outport  Port=2
  wires:
  FFT_estimation/2(phase) -> phase/1
  FFT_estimation/1(amp) -> amp/1
  u/1 -> Sampling/1
  Constant4/1 -> FFT_estimation/3(f0)
  Constant5/1 -> FFT_estimation/2(fs)
  Buffer 10cycle/1 -> FFT_estimation/1(u)
  Sampling/1 -> Buffer 10cycle/1

== matlab function CoSimV1/PFC Control/fft estimation 1 cycle2/FFT_estimation_1 ==
  data: u input; amp output; phase output; fs input; f0 input
function [amp, phase] = FFT_estimation_1(u, fs, f0)
%#codegen

x = double(u(:));
N = length(x);

h = zeros(4, 1);
h(1) = 1;
h(2) = 3;
h(3) = 5;
h(4) = 7;

X = fft(x);

amp = zeros(4, 1);
phase_abs_sin = zeros(4, 1);
phase = zeros(3, 1);

tol = 1e-12;

for i = 1:4
    harmonicOrder = h(i);

    bin = round(harmonicOrder * f0 * double(N) / fs);

    if bin <= 0 || bin > floor(double(N) / 2)
        amp(i) = 0;
        phase_abs_sin(i) = 0;
    else
        idx = int32(bin + 1);
        C = X(idx);

        if mod(N, 2) == 0 && bin == N / 2
            amp(i) = abs(C) / double(N);
        else
            amp(i) = 2 * abs(C) / double(N);
        end

        if amp(i) < tol
            phase_abs_sin(i) = 0;
        else
            ph_raw = angle(C);

            ph_sin = ph_raw + pi/2;

            phase_abs_sin(i) = atan2(sin(ph_sin), cos(ph_sin));
        end
    end
end

if amp(1) < tol
    phase(1) = 0;
    phase(2) = 0;
    phase(3) = 0;
else
    phase(1) = atan2( ...
        sin(phase_abs_sin(2) - 3 * phase_abs_sin(1)), ...
        cos(phase_abs_sin(2) - 3 * phase_abs_sin(1)) ...
    );

    phase(2) = atan2( ...
        sin(phase_abs_sin(3) - 5 * phase_abs_sin(1)), ...
        cos(phase_abs_sin(3) - 5 * phase_abs_sin(1)) ...
    );

    phase(3) = atan2( ...
        sin(phase_abs_sin(4) - 7 * phase_abs_sin(1)), ...
        cos(phase_abs_sin(4) - 7 * phase_abs_sin(1)) ...
    );
end

end

== matlab function CoSimV1/PFC Control/fft estimation 10 cycle2/FFT_estimation ==
  data: u input; amp output; phase output; fs input; f0 input
function [amp, phase] = FFT_estimation(u, fs, f0)
%#codegen

x = double(u(:));
N = length(x);

h = zeros(4, 1);
h(1) = 1;
h(2) = 3;
h(3) = 5;
h(4) = 7;

X = fft(x);

amp = zeros(4, 1);
phase_abs_sin = zeros(4, 1);
phase = zeros(3, 1);

tol = 1e-12;

for i = 1:4
    harmonicOrder = h(i);

    bin = round(harmonicOrder * f0 * double(N) / fs);

    if bin <= 0 || bin > floor(double(N) / 2)
        amp(i) = 0;
        phase_abs_sin(i) = 0;
    else
        idx = int32(bin + 1);
        C = X(idx);

        if mod(N, 2) == 0 && bin == N / 2
            amp(i) = abs(C) / double(N);
        else
            amp(i) = 2 * abs(C) / double(N);
        end

        if amp(i) < tol
            phase_abs_sin(i) = 0;
        else
            ph_raw = angle(C);

            ph_sin = ph_raw + pi/2;

            phase_abs_sin(i) = atan2(sin(ph_sin), cos(ph_sin));
        end
    end
end

if amp(1) < tol
    phase(1) = 0;
    phase(2) = 0;
    phase(3) = 0;
else
    phase(1) = atan2( ...
        sin(phase_abs_sin(2) - 3 * phase_abs_sin(1)), ...
        cos(phase_abs_sin(2) - 3 * phase_abs_sin(1)) ...
    );

    phase(2) = atan2( ...
        sin(phase_abs_sin(3) - 5 * phase_abs_sin(1)), ...
        cos(phase_abs_sin(3) - 5 * phase_abs_sin(1)) ...
    );

    phase(3) = atan2( ...
        sin(phase_abs_sin(4) - 7 * phase_abs_sin(1)), ...
        cos(phase_abs_sin(4) - 7 * phase_abs_sin(1)) ...
    );
end

end

== matlab function CoSimV1/PFC Control/One  Cycle Model Prediction/MATLAB Function ==
  data: x input; x_norm output; A output
function [x_norm, A] = CycleNorm(x)
A = max(abs(x));
A = max(A, 1e-6);
x_norm = x / A;

== matlab function CoSimV1/PFC Control/D_predict ==
  data: i_L input; D output; i_ref input; V_in input; Ts input; L_in input; V_o input; theta_pll input; amp_est input; phase_est input; use_harmonic input
function D  = fcn(i_L, i_ref, V_in, Ts, L_in, V_o, theta_pll, amp_est, phase_est, use_harmonic)

    persistent theta_prev;
    if isempty(theta_prev)
        theta_prev = theta_pll;
    end

    % hyper parameters
    track_gain = 0.35;
    damp_gain = 0.015;

    % Optional
    lead_steps = 1.0;


    % Initialisation 
    L = max(L_in, 1e-9);
    Ts_eff = max(Ts, 1e-9);
    Vo = max(abs(V_o), 1.0);
    ui_L = abs(i_L);

    if V_in > 0
        line_sign = 1.0;
    else
        line_sign = -1.0;
    end

    i_ref_signed = line_sign * abs(i_ref);

    plant_gain = line_sign * L / (Vo * Ts_eff);
    D_ff = 1.0 - abs(V_in) / Vo;

    if use_harmonic

        dtheta = atan2(sin(theta_pll - theta_prev), cos(theta_pll - theta_prev));
        theta_prev = theta_pll;

        omega_inst = dtheta / Ts_eff;

        theta_ctrl = theta_pll + omega_inst * Ts_eff * lead_steps;

        A3 = abs(amp_est(2));
        A5 = abs(amp_est(3));
        A7 = abs(amp_est(4));

        phi3 = phase_est(1);
        phi5 = phase_est(2);
        phi7 = phase_est(3);

        phase_sign = 1.0;

        ih3 = A3 * sin(3.0 * theta_ctrl + phase_sign * phi3);
        ih5 = A5 * sin(5.0 * theta_ctrl + phase_sign * phi5);
        ih7 = A7 * sin(7.0 * theta_ctrl + phase_sign * phi7);

        k3 = 1.00;
        k5 = 1.08;
        k7 = 1.00;

        ih_357 = k3 * ih3 + k5 * ih5 + k7 * ih7;

        i_ref_signed = i_ref_signed - ih_357;
    end

    i_err = i_ref_signed - i_L;

    D_corr = plant_gain * track_gain * i_err;
    D_damp = -line_sign * damp_gain * (i_L - i_ref_signed) / ui_L;

    D = D_ff + D_corr + D_damp;
end

== matlab function CoSimV1/PFC Control/UMPC Function Full bridge1 ==
  data: i_L input; y output; i_ref input; V_in input; Ts input; L_in input; V_o input; g_on output; g_off output
function [y,g_on,g_off]= fcn(i_L, i_ref, V_in, Ts, L_in, V_o)

    L=L_in;

    if V_in >= 0
        i_ref_signed = i_ref;
    else
        i_ref_signed = -i_ref;
    end;

    % -- Positive half Cycle
    if V_in >0
        % --- Candidate 1: Switch ON ---
        g_on  = i_L + (V_in)*Ts/L;
        e_on  = abs(g_on - i_ref_signed);
        
        % --- Candidate 2: Switch OFF ---
        g_off = i_L + (V_in - V_o)*Ts/L;
        e_off = abs(g_off - i_ref_signed);

     % -- Negative half Cycle
    else
        % --- Candidate 1: Switch ON ---
        g_on  = i_L + (V_in)*Ts/L;
        e_on  = abs(g_on - i_ref_signed);

        % --- Candidate 2: Switch OFF ---
        g_off = i_L + (V_in + V_o)*Ts/L;
        e_off = abs(g_off - i_ref_signed);
    end

    % --- MPC Decision: pick action with lower predicted error ---
    if e_on <= e_off
        y = true;
    else
        y = false;
    end

== matlab function CoSimV1/PFC Control/One  Cycle Model Prediction/MATLAB Function3 ==
  data: y_rel input; y_post output; A_latest input; alpha input; reset input
function y_post = harmonic_postprocess(y_rel, A_latest, alpha, reset)
%#codegen
% 一体化后处理：
% 1) EMA 平滑（在相对输出域）
% 2) A 恢复（幅值乘 A）
% 3) atan2 恢复相位（由 cos/sin -> phase）
%
% 输入:
%   y_rel    : 模型输出(10x1 或 1x10)
%              [amp_h1_rel, amp_h3_rel, amp_h5_rel, amp_h7_rel, ...
%               cos_h3, sin_h3, cos_h5, sin_h5, cos_h7, sin_h7]
%   A_latest : A 恢复系数（可标量或向量；向量时自动取 max(abs(.))）
%   alpha    : EMA 系数 [0,1]，建议 0.10~0.16
%   reset    : 复位信号（true 时重置 EMA 状态）
%
% 输出:
%   y_post(7x1):
%   [amp_h1_abs, amp_h3_abs, amp_h5_abs, amp_h7_abs, phase_h3, phase_h5, phase_h7]

persistent ema_state initialized
if isempty(initialized)
    ema_state = zeros(10,1,'single');
    initialized = false;
end

% -------- 参数/输入整理 --------
y = zeros(10,1,'single');
for i = 1:10
    y(i) = single(y_rel(i));
end

a = single(abs(A_latest));
if numel(a) > 1
    a = max(a(:));
end
if a < single(1e-6)
    a = single(1e-6);
end

a_ema = single(alpha);
if a_ema < single(0)
    a_ema = single(0);
elseif a_ema > single(1)
    a_ema = single(1);
end

do_reset = (reset ~= 0);

% -------- EMA --------
if ~initialized || do_reset
    ema_state = y;
    initialized = true;
else
    ema_state = a_ema * y + (single(1) - a_ema) * ema_state;
end

% -------- A 恢复（幅值）--------
amp = ema_state(1:4) * a;

% -------- 相位恢复（cos/sin -> atan2）--------
% 先单位化，避免 cos/sin 长度漂移导致相位抖动
c3 = ema_state(5); s3 = ema_state(6);
n3 = sqrt(c3*c3 + s3*s3); if n3 < single(1e-6), n3 = single(1e-6); end
c3 = c3 / n3; s3 = s3 / n3;

c5 = ema_state(7); s5 = ema_state(8);
n5 = sqrt(c5*c5 + s5*s5); if n5 < single(1e-6), n5 = single(1e-6); end
c5 = c5 / n5; s5 = s5 / n5;

c7 = ema_state(9); s7 = ema_state(10);
n7 = sqrt(c7*c7 + s7*s7); if n7 < single(1e-6), n7 = single(1e-6); end
c7 = c7 / n7; s7 = s7 / n7;

ph3 = atan2(s3, c3);
ph5 = atan2(s5, c5);
ph7 = atan2(s7, c7);

% -------- 最终输出（仅最终量）--------
y_post = zeros(7,1,'single');
y_post(1:4) = amp;
y_post(5) = ph3;
y_post(6) = ph5;
y_post(7) = ph7;

end

== matlab function CoSimV1/PFC Control/Half Cycle Model Prediction/MATLAB Function ==
  data: x input; x_norm output; A output
function [x_norm, A] = CycleNorm(x)
A = max(abs(x));
A = max(A, 1e-6);
x_norm = x / A;

== matlab function CoSimV1/PFC Control/Half Cycle Model Prediction/MATLAB Function3 ==
  data: y_rel input; y_post output; A_latest input; alpha input; reset input
function y_post = harmonic_postprocess(y_rel, A_latest, alpha, reset)
%#codegen
% 一体化后处理：
% 1) EMA 平滑（在相对输出域）
% 2) A 恢复（幅值乘 A）
% 3) atan2 恢复相位（由 cos/sin -> phase）
%
% 输入:
%   y_rel    : 模型输出(10x1 或 1x10)
%              [amp_h1_rel, amp_h3_rel, amp_h5_rel, amp_h7_rel, ...
%               cos_h3, sin_h3, cos_h5, sin_h5, cos_h7, sin_h7]
%   A_latest : A 恢复系数（可标量或向量；向量时自动取 max(abs(.))）
%   alpha    : EMA 系数 [0,1]，建议 0.10~0.16
%   reset    : 复位信号（true 时重置 EMA 状态）
%
% 输出:
%   y_post(7x1):
%   [amp_h1_abs, amp_h3_abs, amp_h5_abs, amp_h7_abs, phase_h3, phase_h5, phase_h7]

persistent ema_state initialized
if isempty(initialized)
    ema_state = zeros(10,1,'single');
    initialized = false;
end

% -------- 参数/输入整理 --------
y = zeros(10,1,'single');
for i = 1:10
    y(i) = single(y_rel(i));
end

a = single(abs(A_latest));
if numel(a) > 1
    a = max(a(:));
end
if a < single(1e-6)
    a = single(1e-6);
end

a_ema = single(alpha);
if a_ema < single(0)
    a_ema = single(0);
elseif a_ema > single(1)
    a_ema = single(1);
end

do_reset = (reset ~= 0);

% -------- EMA --------
if ~initialized || do_reset
    ema_state = y;
    initialized = true;
else
    ema_state = a_ema * y + (single(1) - a_ema) * ema_state;
end

% -------- A 恢复（幅值）--------
amp = ema_state(1:4) * a;

% -------- 相位恢复（cos/sin -> atan2）--------
% 先单位化，避免 cos/sin 长度漂移导致相位抖动
c3 = ema_state(5); s3 = ema_state(6);
n3 = sqrt(c3*c3 + s3*s3); if n3 < single(1e-6), n3 = single(1e-6); end
c3 = c3 / n3; s3 = s3 / n3;

c5 = ema_state(7); s5 = ema_state(8);
n5 = sqrt(c5*c5 + s5*s5); if n5 < single(1e-6), n5 = single(1e-6); end
c5 = c5 / n5; s5 = s5 / n5;

c7 = ema_state(9); s7 = ema_state(10);
n7 = sqrt(c7*c7 + s7*s7); if n7 < single(1e-6), n7 = single(1e-6); end
c7 = c7 / n7; s7 = s7 / n7;

ph3 = atan2(s3, c3);
ph5 = atan2(s5, c5);
ph7 = atan2(s7, c7);

% -------- 最终输出（仅最终量）--------
y_post = zeros(7,1,'single');
y_post(1:4) = amp;
y_post(5) = ph3;
y_post(6) = ph5;
y_post(7) = ph7;

end

== matlab function CoSimV1/PFC Control/MCP Function Half bridge1 ==
  data: i_L input; y output; i_ref input; V_in input; Ts input; L_in input; V_o input
function y = fcn(i_L, i_ref, V_in, Ts, L_in, V_o)

    L=2*pi*50*L_in;
    % --- Candidate 1: Switch ON ---
    g_on  = i_L + abs(V_in)*Ts/L;
    e_on  = abs(g_on - i_ref);

    % --- Candidate 2: Switch OFF ---
    g_off = i_L + (abs(V_in)-V_o)*Ts/L;
    e_off = abs(g_off - i_ref);

    % --- MPC Decision: pick action with lower predicted error ---
    if e_on <= e_off
        y = true;
    else
        y = false;
    end

== matlab function CoSimV1/PFC Control/RLS_estimation ==
  data: i_L input; amp_est output; theta_pll input; Ts input; reset input; phase_est output; i_h_est output; thdi_est output
function [amp_est, phase_est, i_h_est, thdi_est] = RLS_estimation(i_L, theta_pll, Ts, reset)
%#codegen

nParam = 9;

amp_est = zeros(4, 1);
phase_est = zeros(3, 1);
i_h_est = 0.0;
thdi_est = 0.0;

Ts_eff = max(Ts, 1e-9);

persistent w;
persistent wf;
persistent P;
persistent Ipk_filt;
persistent phase_prev;

if isempty(w) || reset ~= 0
    w = zeros(nParam, 1);
    wf = zeros(nParam, 1);
    P = zeros(nParam, nParam);

    P0 = 250.0;

    for r = 1:nParam
        for c = 1:nParam
            if r == c
                P(r, c) = P0;
            else
                P(r, c) = 0.0;
            end
        end
    end

    Ipk_filt = max(abs(i_L), 1.0);
    phase_prev = zeros(3, 1);
end

Ipk_guard = max(Ipk_filt, 1.0);

tau_est = 0.018;
lambda = exp(-Ts_eff / tau_est);

if lambda < 0.980
    lambda = 0.980;
elseif lambda > 0.99998
    lambda = 0.99998;
end

theta = atan2(sin(theta_pll), cos(theta_pll));

s1 = sin(theta);
c1 = cos(theta);

s3 = sin(3.0 * theta);
c3 = cos(3.0 * theta);

s5 = sin(5.0 * theta);
c5 = cos(5.0 * theta);

s7 = sin(7.0 * theta);
c7 = cos(7.0 * theta);

x = zeros(nParam, 1);

x(1) = 1.0;
x(2) = s1;
x(3) = c1;
x(4) = s3;
x(5) = c3;
x(6) = s5;
x(7) = c5;
x(8) = s7;
x(9) = c7;

y_hat = 0.0;

for k = 1:nParam
    y_hat = y_hat + x(k) * w(k);
end

e = i_L - y_hat;

e_lim = 0.25 * Ipk_guard;

if e_lim < 0.5
    e_lim = 0.5;
end

if e > e_lim
    e = e_lim;
elseif e < -e_lim
    e = -e_lim;
end

Px = zeros(nParam, 1);

for r = 1:nParam
    acc = 0.0;

    for c = 1:nParam
        acc = acc + P(r, c) * x(c);
    end

    Px(r) = acc;
end

xTPx = 0.0;

for k = 1:nParam
    xTPx = xTPx + x(k) * Px(k);
end

den = lambda + xTPx;

if den < 1e-9
    den = 1e-9;
end

K = zeros(nParam, 1);

for k = 1:nParam
    K(k) = Px(k) / den;
end

for k = 1:nParam
    w(k) = w(k) + K(k) * e;
end

for r = 1:nParam
    for c = 1:nParam
        P(r, c) = (P(r, c) - K(r) * Px(c)) / lambda;
    end
end

for r = 1:nParam
    for c = 1:nParam
        if c > r
            p_avg = 0.5 * (P(r, c) + P(c, r));
            P(r, c) = p_avg;
            P(c, r) = p_avg;
        end
    end
end

Pmax = 1e5;
Pmin = 1e-7;

for k = 1:nParam
    if P(k, k) > Pmax
        P(k, k) = Pmax;
    elseif P(k, k) < Pmin
        P(k, k) = Pmin;
    end
end

tau_out = 0.004;
alpha_w = 1.0 - exp(-Ts_eff / tau_out);

if alpha_w < 0.001
    alpha_w = 0.001;
elseif alpha_w > 0.10
    alpha_w = 0.10;
end

for k = 1:nParam
    wf(k) = (1.0 - alpha_w) * wf(k) + alpha_w * w(k);
end

a1 = wf(2);
b1 = wf(3);

a3 = wf(4);
b3 = wf(5);

a5 = wf(6);
b5 = wf(7);

a7 = wf(8);
b7 = wf(9);

A1 = sqrt(a1 * a1 + b1 * b1);
A3 = sqrt(a3 * a3 + b3 * b3);
A5 = sqrt(a5 * a5 + b5 * b5);
A7 = sqrt(a7 * a7 + b7 * b7);

Ipk_now = max(abs(i_L), A1);

if Ipk_now > Ipk_filt
    Ipk_filt = 0.05 * Ipk_now + 0.95 * Ipk_filt;
else
    Ipk_filt = 0.002 * Ipk_now + 0.998 * Ipk_filt;
end

Ipk = max(Ipk_filt, 1e-6);

A1_lim = 1.50 * Ipk;
A3_lim = 0.20 * Ipk;
A5_lim = 0.20 * Ipk;
A7_lim = 0.20 * Ipk;

if A1 > A1_lim
    A1 = A1_lim;
end

if A3 > A3_lim
    A3 = A3_lim;
end

if A5 > A5_lim
    A5 = A5_lim;
end

if A7 > A7_lim
    A7 = A7_lim;
end

phase_min = 0.0015 * Ipk;

if A3 > phase_min
    phi3 = atan2(b3, a3);
    phase_prev(1) = phi3;
else
    phi3 = phase_prev(1);
end

if A5 > phase_min
    phi5 = atan2(b5, a5);
    phase_prev(2) = phi5;
else
    phi5 = phase_prev(2);
end

if A7 > phase_min
    phi7 = atan2(b7, a7);
    phase_prev(3) = phi7;
else
    phi7 = phase_prev(3);
end

phi3 = atan2(sin(phi3), cos(phi3));
phi5 = atan2(sin(phi5), cos(phi5));
phi7 = atan2(sin(phi7), cos(phi7));

amp_est(1) = A1;
amp_est(2) = A3;
amp_est(3) = A5;
amp_est(4) = A7;

phase_est(1) = phi3;
phase_est(2) = phi5;
phase_est(3) = phi7;

i_h_est = a3 * s3 + b3 * c3 + a5 * s5 + b5 * c5 + a7 * s7 + b7 * c7;

if A1 > 1e-6
    thdi_est = sqrt(A3 * A3 + A5 * A5 + A7 * A7) / A1;
else
    thdi_est = 0.0;
end

end
